simulink model "obserwator_2"  (R2023b)
settings: Solver=VariableStepAuto  StartTime=0.0  StopTime=10.0  RelTol=1e-3
values from neighbouring files (symbols this model uses):
  k = acker(A, B, [s_b s_b s_b])    [obiekt.m]
  L = acker(A', C', [s_0, s_0, s_0])'    [obiekt.m]
undefined symbols (not defined in the file or in its folder): C
settings Model: Creator=pavig  LastModifiedBy=pavig

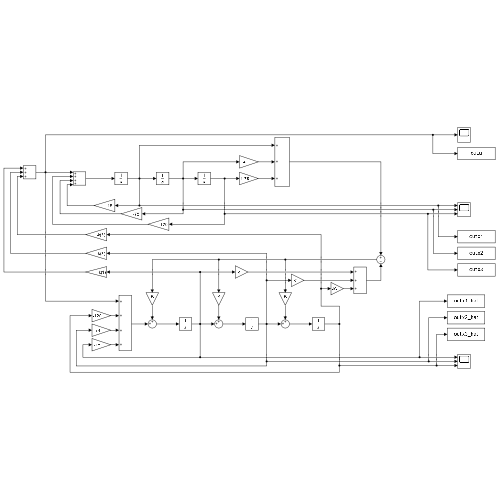
[thumbnail: Simulink's stored preview of the top-level diagram]
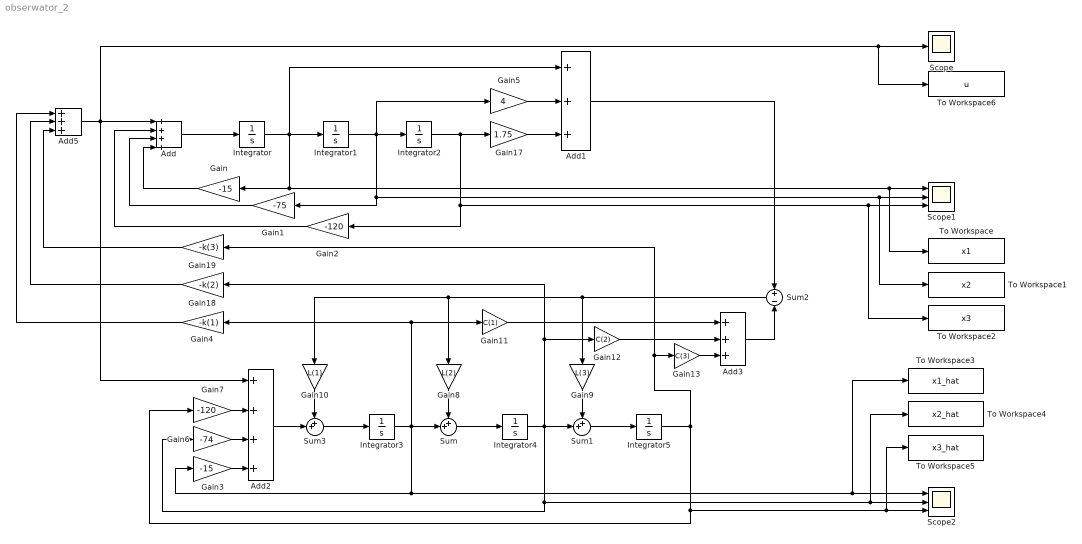
== system obserwator_2 ==
  Add : Sum  Inputs=++++
  Add1 : Sum  Inputs=+++
  Add2 : Sum  Inputs=++++
  Add3 : Sum  Inputs=+++
  Add5 : Sum  Inputs=+++
  Gain : Gain  Gain=-15
  Gain1 : Gain  Gain=-75
  Gain10 : Gain  Gain=L(1)
  Gain11 : Gain  Gain=C(1)
  Gain12 : Gain  Gain=C(2)
  Gain13 : Gain  Gain=C(3)
  Gain17 : Gain  Gain=1.75
  Gain18 : Gain  Gain=-k(2)
  Gain19 : Gain  Gain=-k(3)
  Gain2 : Gain  Gain=-120
  Gain3 : Gain  Gain=-15
  Gain4 : Gain  Gain=-k(1)
  Gain5 : Gain  Gain=4
  Gain6 : Gain  Gain=-74
  Gain7 : Gain  Gain=-120
  Gain8 : Gain  Gain=L(2)
  Gain9 : Gain  Gain=L(3)
  Integrator : Integrator  InitialCondition=-1
  Integrator1 : Integrator  InitialCondition=2
  Integrator2 : Integrator  InitialCondition=1
  Integrator3 : Integrator
  Integrator4 : Integrator
  Integrator5 : Integrator
  Scope : Scope
  Scope1 : Scope  NumInputPorts=3
  Scope2 : Scope  NumInputPorts=3
  Sum : Sum  Inputs=++|
  Sum1 : Sum  Inputs=++|
  Sum2 : Sum  Inputs=+-
  Sum3 : Sum  Inputs=++|
  To Workspace : ToWorkspace  VariableName=x1  SaveFormat=Timeseries  SampleTime=-1
  To Workspace1 : ToWorkspace  VariableName=x2  SaveFormat=Timeseries  SampleTime=-1
  To Workspace2 : ToWorkspace  VariableName=x3  SaveFormat=Timeseries  SampleTime=-1
  To Workspace3 : ToWorkspace  VariableName=x1_hat  SaveFormat=Timeseries  SampleTime=-1
  To Workspace4 : ToWorkspace  VariableName=x2_hat  SaveFormat=Timeseries  SampleTime=-1
  To Workspace5 : ToWorkspace  VariableName=x3_hat  SaveFormat=Timeseries  SampleTime=-1
  To Workspace6 : ToWorkspace  VariableName=u  SaveFormat=Timeseries  SampleTime=-1
  wires:
  Add2/1 -> Sum3/2
  Sum3/1 -> Integrator3/1
  Add3/1 -> Sum2/2
  Sum2/1 -> Gain9/1, Gain8/1, Gain10/1
  Gain3/1 -> Add2/4
  Gain11/1 -> Add3/1
  Gain9/1 -> Sum1/1
  Integrator5/1 -> Gain7/1, To Workspace5/1, Scope2/3, Gain19/1, Gain13/1
  Sum/1 -> Integrator4/1
  Gain13/1 -> Add3/3
  Integrator2/1 -> Gain17/1, Gain2/1, Scope1/3, To Workspace2/1
  Add/1 -> Integrator/1
  Integrator4/1 -> Sum1/2, Gain6/1, To Workspace4/1, Scope2/2, Gain18/1, Gain12/1
  Add1/1 -> Sum2/1
  Gain10/1 -> Sum3/1
  Gain/1 -> Add/4
  Add5/1 -> Add2/1, To Workspace6/1, Scope/1, Add/1
  Integrator1/1 -> Gain5/1, Gain1/1, To Workspace1/1, Scope1/2, Integrator2/1
  Integrator/1 -> Add1/1, Gain/1, Scope1/1, To Workspace/1, Integrator1/1
  Gain2/1 -> Add/2
  Gain6/1 -> Add2/3
  Gain12/1 -> Add3/2
  Gain17/1 -> Add1/3
  Gain7/1 -> Add2/2
  Gain1/1 -> Add/3
  Gain5/1 -> Add1/2
  Integrator3/1 -> Sum/2, Gain3/1, To Workspace3/1, Scope2/1, Gain4/1, Gain11/1
  Gain8/1 -> Sum/1
  Sum1/1 -> Integrator5/1
  Gain19/1 -> Add5/3
  Gain18/1 -> Add5/2
  Gain4/1 -> Add5/1
